simulink model "AOs_sim"  (R2024a)
settings: Solver=ode1  StartTime=0.0  StopTime=inf  FixedStep=0.002  RelTol=1e-3
(part 1 of 2)
settings Model: Creator=Enrica Tricomi  LastModifiedBy=tsmoragiewicz
settings OptimizationCC: ReuseModelBlockBuffer=off
settings RTWCC: GPUComputeCapability=3.5

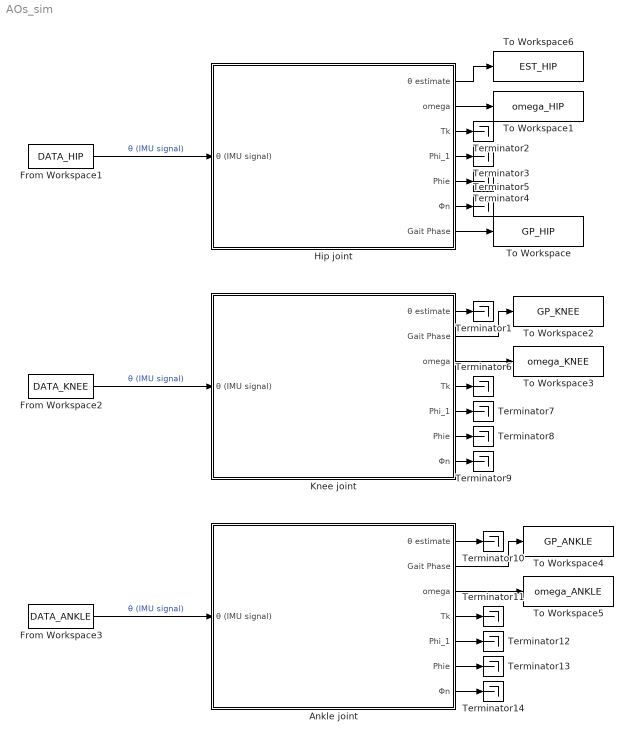
== system AOs_sim ==
  Ankle joint : Subsystem
  From Workspace1 : FromWorkspace  VariableName=DATA_HIP  SampleTime=-1
  From Workspace2 : FromWorkspace  VariableName=DATA_KNEE  SampleTime=-1
  From Workspace3 : FromWorkspace  VariableName=DATA_ANKLE  SampleTime=-1
  Hip joint : Subsystem
  Knee joint : Subsystem
  Terminator{1..14} (14 alike) : Terminator
  To Workspace : ToWorkspace  VariableName=GP_HIP  SampleTime=-1
  To Workspace1 : ToWorkspace  VariableName=omega_HIP  SampleTime=-1
  To Workspace2 : ToWorkspace  VariableName=GP_KNEE  SampleTime=-1
  To Workspace3 : ToWorkspace  VariableName=omega_KNEE  SampleTime=-1
  To Workspace4 : ToWorkspace  VariableName=GP_ANKLE  SampleTime=-1
  To Workspace5 : ToWorkspace  VariableName=omega_ANKLE  SampleTime=-1
  To Workspace6 : ToWorkspace  VariableName=EST_HIP  SampleTime=-1
  wires:
  Hip joint/4(Phi_1) -> Terminator3/1
  Hip joint/3(Tk) -> Terminator2/1
  Hip joint/1(θ estimate) -> To Workspace6/1
  Hip joint/6(Φn) -> Terminator5/1
  Hip joint/7(Gait Phase) -> To Workspace/1
  Hip joint/5(Phie) -> Terminator4/1
  Hip joint/2(omega) -> To Workspace1/1
  From Workspace1/1 -> Hip joint/1(θ (IMU signal))  "θ (IMU signal)"
  Knee joint/5(Phi_1) -> Terminator7/1
  Knee joint/4(Tk) -> Terminator6/1
  Knee joint/7(Φn) -> Terminator9/1
  Knee joint/2(Gait Phase) -> To Workspace2/1
  Knee joint/6(Phie) -> Terminator8/1
  Knee joint/3(omega) -> To Workspace3/1
  Knee joint/1(θ estimate) -> Terminator1/1
  Ankle joint/2(Gait Phase) -> To Workspace4/1
  Ankle joint/3(omega) -> To Workspace5/1
  Ankle joint/6(Phie) -> Terminator13/1
  Ankle joint/7(Φn) -> Terminator14/1
  Ankle joint/4(Tk) -> Terminator11/1
  Ankle joint/5(Phi_1) -> Terminator12/1
  Ankle joint/1(θ estimate) -> Terminator10/1
  From Workspace3/1 -> Ankle joint/1(θ (IMU signal))  "θ (IMU signal)"
  From Workspace2/1 -> Knee joint/1(θ (IMU signal))  "θ (IMU signal)"

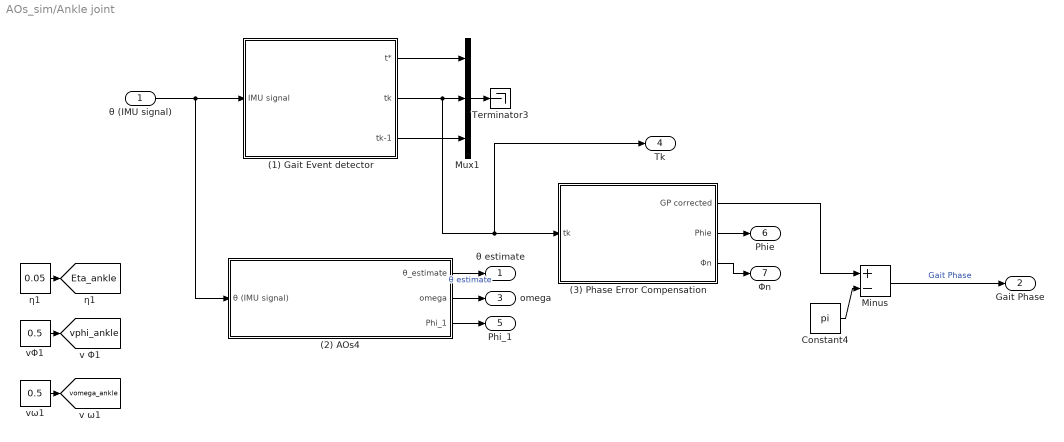
== system AOs_sim/Ankle joint ==
  θ (IMU signal) : Inport
  (1) Gait Event detector : Subsystem
  (2) AOs4 : Subsystem
  (3) Phase Error Compensation : Subsystem
  Constant4 : Constant  Value=pi
  Minus : Sum  Inputs=+-
  Mux1 : Mux  Inputs=3
  Terminator3 : Terminator
  vΦ1 : Constant  Value=0.5
  vω1 : Constant  Value=0.5
  η1 : Constant  Value=0.05
  θ estimate : Outport
  Gait Phase : Outport  Port=2
  omega : Outport  Port=3
  Tk : Outport  Port=4
  Phi_1 : Outport  Port=5
  Phie : Outport  Port=6
  Φn : Outport  Port=7
  tag scope: Eta_ankle=global, vomega_ankle=global, vphi_ankle=global
  wires:
  Constant4/1 -> Minus/2
  Mux1/1 -> Terminator3/1
  (2) AOs4/1(θ_estimate) -> θ estimate/1  "θ estimate"
  (1) Gait Event detector/3(tk-1) -> Mux1/3
  (1) Gait Event detector/1(t*) -> Mux1/1
  θ (IMU signal)/1 -> (1) Gait Event detector/1(IMU signal), (2) AOs4/1(θ (IMU signal))
  (3) Phase Error Compensation/1(GP corrected) -> Minus/1
  Minus/1 -> Gait Phase/1  "Gait Phase"
  (2) AOs4/2(omega) -> omega/1
  (1) Gait Event detector/2(tk) -> Tk/1, (3) Phase Error Compensation/1(tk), Mux1/2
  (2) AOs4/3(Phi_1) -> Phi_1/1
  (3) Phase Error Compensation/2(Phie) -> Phie/1
  (3) Phase Error Compensation/3(Φn) -> Φn/1
  vΦ1/1 -> [vphi_ankle]
  vω1/1 -> [vomega_ankle]
  η1/1 -> [Eta_ankle]

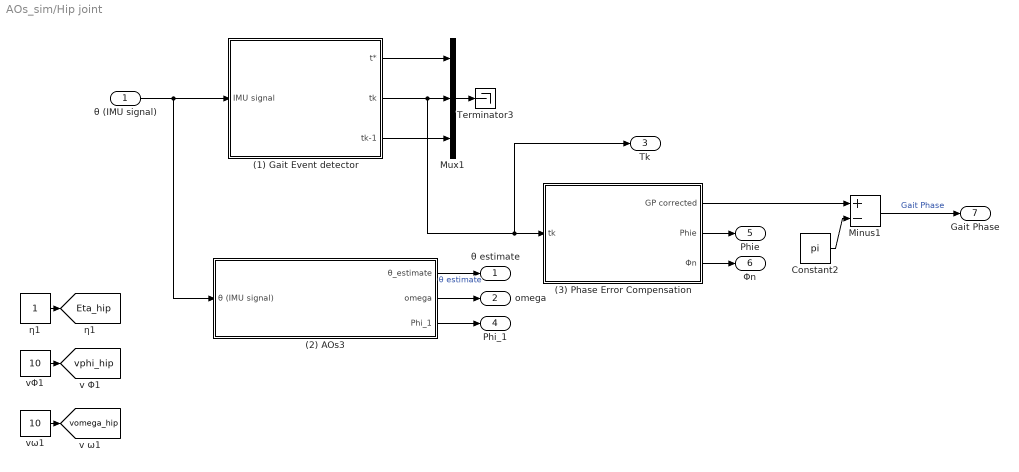
== system AOs_sim/Hip joint ==
  θ (IMU signal) : Inport
  (1) Gait Event detector : Subsystem
  (2) AOs3 : Subsystem
  (3) Phase Error Compensation : Subsystem
  Constant2 : Constant  Value=pi
  Minus1 : Sum  Inputs=+-
  Mux1 : Mux  Inputs=3
  Terminator3 : Terminator
  vΦ1 : Constant  Value=10
  vω1 : Constant  Value=10
  η1 : Constant
  θ estimate : Outport
  omega : Outport  Port=2
  Tk : Outport  Port=3
  Phi_1 : Outport  Port=4
  Phie : Outport  Port=5
  Φn : Outport  Port=6
  Gait Phase : Outport  Port=7
  tag scope: Eta_hip=global, vomega_hip=global, vphi_hip=global
  wires:
  Mux1/1 -> Terminator3/1
  (2) AOs3/1(θ_estimate) -> θ estimate/1  "θ estimate"
  (1) Gait Event detector/3(tk-1) -> Mux1/3
  (1) Gait Event detector/1(t*) -> Mux1/1
  (2) AOs3/2(omega) -> omega/1
  (1) Gait Event detector/2(tk) -> Tk/1, (3) Phase Error Compensation/1(tk), Mux1/2
  (3) Phase Error Compensation/2(Phie) -> Phie/1
  (3) Phase Error Compensation/3(Φn) -> Φn/1
  (2) AOs3/3(Phi_1) -> Phi_1/1
  Constant2/1 -> Minus1/2
  (3) Phase Error Compensation/1(GP corrected) -> Minus1/1
  Minus1/1 -> Gait Phase/1  "Gait Phase"
  θ (IMU signal)/1 -> (1) Gait Event detector/1(IMU signal), (2) AOs3/1(θ (IMU signal))
  vΦ1/1 -> [vphi_hip]
  vω1/1 -> [vomega_hip]
  η1/1 -> [Eta_hip]

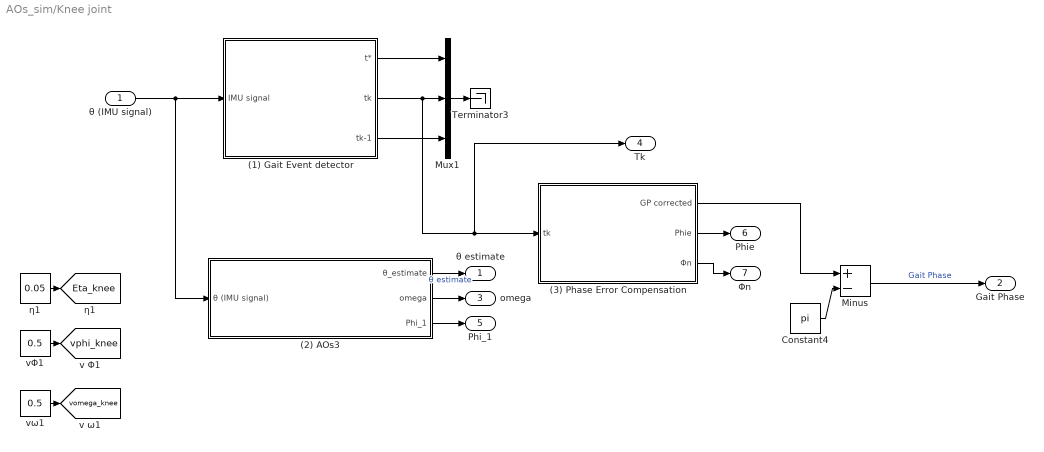
== system AOs_sim/Knee joint ==
  θ (IMU signal) : Inport
  (1) Gait Event detector : Subsystem
  (2) AOs3 : Subsystem
  (3) Phase Error Compensation : Subsystem
  Constant4 : Constant  Value=pi
  Minus : Sum  Inputs=+-
  Mux1 : Mux  Inputs=3
  Terminator3 : Terminator
  vΦ1 : Constant  Value=0.5
  vω1 : Constant  Value=0.5
  η1 : Constant  Value=0.05
  θ estimate : Outport
  Gait Phase : Outport  Port=2
  omega : Outport  Port=3
  Tk : Outport  Port=4
  Phi_1 : Outport  Port=5
  Phie : Outport  Port=6
  Φn : Outport  Port=7
  tag scope: Eta_knee=global, vomega_knee=global, vphi_knee=global
  wires:
  Constant4/1 -> Minus/2
  Mux1/1 -> Terminator3/1
  (2) AOs3/1(θ_estimate) -> θ estimate/1  "θ estimate"
  (1) Gait Event detector/3(tk-1) -> Mux1/3
  (1) Gait Event detector/1(t*) -> Mux1/1
  θ (IMU signal)/1 -> (1) Gait Event detector/1(IMU signal), (2) AOs3/1(θ (IMU signal))
  (3) Phase Error Compensation/1(GP corrected) -> Minus/1
  Minus/1 -> Gait Phase/1  "Gait Phase"
  (2) AOs3/2(omega) -> omega/1
  (1) Gait Event detector/2(tk) -> Tk/1, (3) Phase Error Compensation/1(tk), Mux1/2
  (2) AOs3/3(Phi_1) -> Phi_1/1
  (3) Phase Error Compensation/2(Phie) -> Phie/1
  (3) Phase Error Compensation/3(Φn) -> Φn/1
  η1/1 -> [Eta_knee]
  vω1/1 -> [vomega_knee]
  vΦ1/1 -> [vphi_knee]

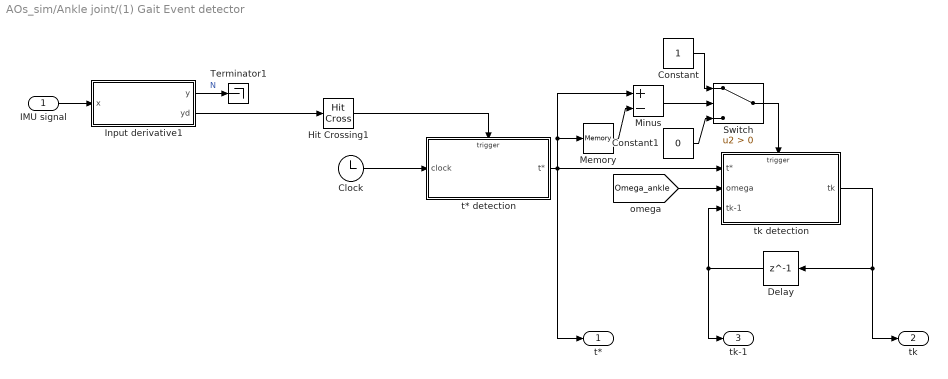
== system AOs_sim/Ankle joint/(1) Gait Event detector ==
  IMU signal : Inport
  Clock : Clock
  Constant : Constant
  Constant1 : Constant  Value=0
  Delay : Delay  DelayLength=1
  Hit Crossing1 : HitCross  HitCrossingOffset=0.2  HitCrossingDirection=falling
  Input derivative1 : Subsystem  mask{wn=40, zt=1, x0=0}
      mask prompts: wn "Cut-off frequency (rad/s)"; zt "Damping ratio"; x0 "Initial Condition"
      mask Display: disp('Second-Order\nLow-Pass Filter');
  Memory : Memory
  Minus : Sum  Inputs=+-
  Switch : Switch  Criteria=u2 > Threshold  SaturateOnIntegerOverflow=off  InputSameDT=off
  Terminator1 : Terminator
  t* detection : Subsystem
  tk detection : Subsystem
  t* : Outport
  tk : Outport  Port=2
  tk-1 : Outport  Port=3
  wires:
  Clock/1 -> t* detection/1(clock)
  Hit Crossing1/1 -> t* detection/Trigger
  t* detection/1(t*) -> tk detection/1(t*), t*/1, Minus/1, Memory/1
  [Omega_ankle] -> tk detection/2(omega)
  Constant/1 -> Switch/1
  Constant1/1 -> Switch/3
  Minus/1 -> Switch/2
  Memory/1 -> Minus/2
  Switch/1 -> tk detection/Trigger
  Delay/1 -> tk detection/3(tk-1), tk-1/1
  tk detection/1(tk) -> tk/1, Delay/1
  Input derivative1/2(yd) -> Hit Crossing1/1
  IMU signal/1 -> Input derivative1/1(x)
  Input derivative1/1(y) -> Terminator1/1  "N"

== system AOs_sim/Ankle joint/(2) AOs4 ==
  note: Pool of Adaptive Oscillators
  θ (IMU signal) : Inport
  AO0 : Subsystem
  AO1 : Subsystem
  AO2 : Subsystem
  AO3 : Subsystem
  AO4 : Subsystem
  AO5 : Subsystem
  Sum : Sum  Inputs=|+-
  Sum1 : Sum  Inputs=6
  θ_estimate : Outport
  omega : Outport  Port=2
  Phi_1 : Outport  Port=3
  tag scope: Ft_ankle=global
  wires:
  AO0/1(α0) -> Sum1/1
  Sum1/1 -> θ_estimate/1, Sum/2  "θ_estimate"
  AO4/1(θ_est3) -> Sum1/6
  AO1/1(θ_est1) -> Sum1/2
  Sum/1 -> [Ft_ankle]
  AO2/1(θ_est2) -> Sum1/3
  θ (IMU signal)/1 -> Sum/1
  AO4/2(omega) -> omega/1
  AO1/2(Phi_1) -> Phi_1/1
  AO3/1(θ_est2) -> Sum1/4
  AO5/1(θ_est2) -> Sum1/5

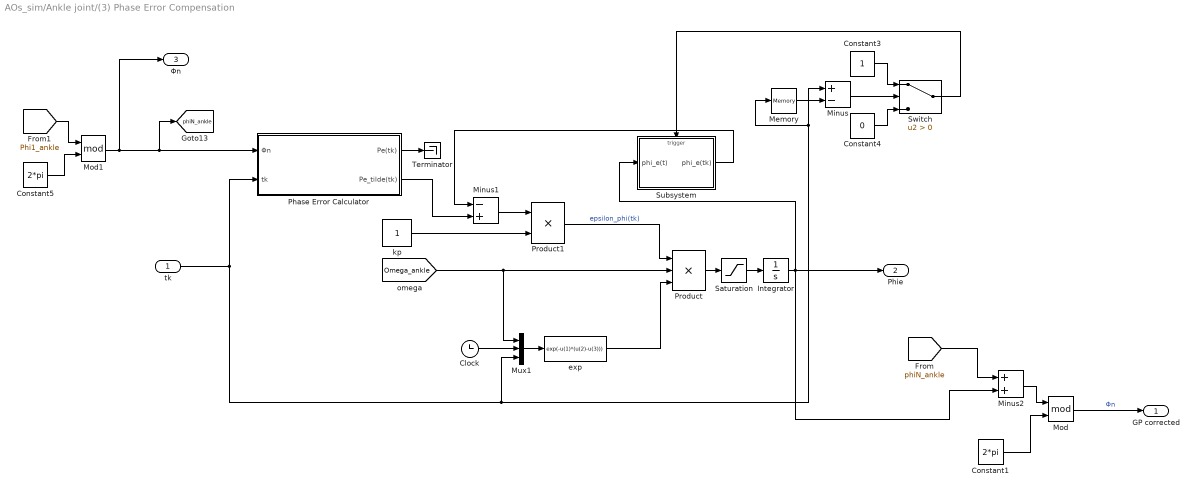
== system AOs_sim/Ankle joint/(3) Phase Error Compensation ==
  tk : Inport
  Clock : Clock
  Constant1 : Constant  Value=2*pi
  Constant3 : Constant
  Constant4 : Constant  Value=0
  Constant5 : Constant  Value=2*pi
  Integrator : Integrator  InitialCondition=0.01
  Memory : Memory
  Minus : Sum  Inputs=+-
  Minus1 : Sum  Inputs=-+
  Minus2 : Sum
  Mod : Math  Operator=mod
  Mod1 : Math  Operator=mod
  Mux1 : Mux  Inputs=3
  Phase Error Calculator : Subsystem
  Product : Product  Inputs=3
  Product1 : Product
  Saturation : Saturate  UpperLimit=10^10  LowerLimit=-10^10
  Subsystem : Subsystem
  Switch : Switch  Criteria=u2 > Threshold  SaturateOnIntegerOverflow=off  InputSameDT=off
  Terminator : Terminator
  exp : Fcn  Expr=exp(-u(1)*(u(2)-u(3)))
  kp : Constant
  GP corrected : Outport
  Phie : Outport  Port=2
  Φn : Outport  Port=3
  tag scope: phiN_ankle=global
  wires:
  Integrator/1 -> Minus2/2, Phie/1, Subsystem/1(phi_e(t))
  Constant1/1 -> Mod/2
  Mux1/1 -> exp/1
  Clock/1 -> Mux1/2
  [phiN_ankle] -> Minus2/1
  [Phi1_ankle] -> Mod1/1
  Product/1 -> Saturation/1
  Minus2/1 -> Mod/1
  Minus1/1 -> Product1/1
  kp/1 -> Product1/2
  Product1/1 -> Product/1  "epsilon_phi(tk)"
  Phase Error Calculator/2(Pe_tilde(tk)) -> Minus1/2
  [Omega_ankle] -> Mux1/1, Product/2
  exp/1 -> Product/3
  Saturation/1 -> Integrator/1
  Constant3/1 -> Switch/1
  Memory/1 -> Minus/2
  Constant4/1 -> Switch/3
  Minus/1 -> Switch/2
  tk/1 -> Phase Error Calculator/2(tk), Minus/1, Memory/1, Mux1/3
  Switch/1 -> Subsystem/Trigger
  Subsystem/1(phi_e(tk)) -> Minus1/1
  Constant5/1 -> Mod1/2
  Mod/1 -> GP corrected/1  "Φn"
  Mod1/1 -> Φn/1, [phiN_ankle], Phase Error Calculator/1(Φn)
  Phase Error Calculator/1(Pe(tk)) -> Terminator/1

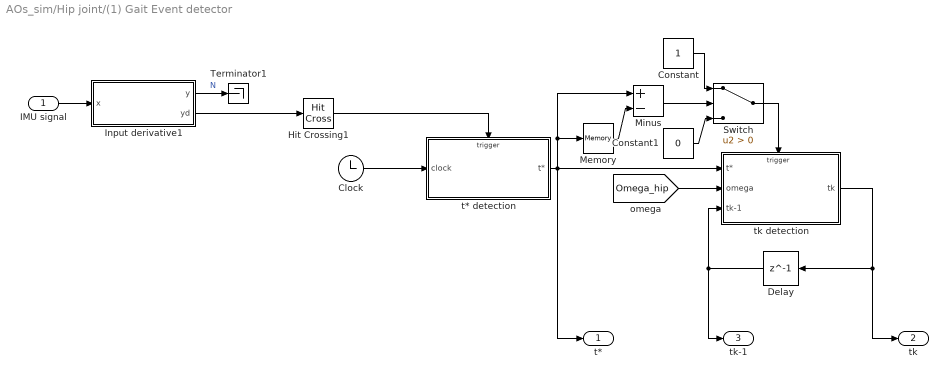
== system AOs_sim/Hip joint/(1) Gait Event detector ==
  IMU signal : Inport
  Clock : Clock
  Constant : Constant
  Constant1 : Constant  Value=0
  Delay : Delay  DelayLength=1
  Hit Crossing1 : HitCross  HitCrossingOffset=0.2  HitCrossingDirection=falling
  Input derivative1 : Subsystem  mask{wn=40, zt=1, x0=0}
      mask prompts: wn "Cut-off frequency (rad/s)"; zt "Damping ratio"; x0 "Initial Condition"
      mask Display: disp('Second-Order\nLow-Pass Filter');
  Memory : Memory
  Minus : Sum  Inputs=+-
  Switch : Switch  Criteria=u2 > Threshold  SaturateOnIntegerOverflow=off  InputSameDT=off
  Terminator1 : Terminator
  t* detection : Subsystem
  tk detection : Subsystem
  t* : Outport
  tk : Outport  Port=2
  tk-1 : Outport  Port=3
  wires:
  Clock/1 -> t* detection/1(clock)
  Hit Crossing1/1 -> t* detection/Trigger
  t* detection/1(t*) -> tk detection/1(t*), t*/1, Minus/1, Memory/1
  [Omega_hip] -> tk detection/2(omega)
  Constant/1 -> Switch/1
  Constant1/1 -> Switch/3
  Minus/1 -> Switch/2
  Memory/1 -> Minus/2
  Switch/1 -> tk detection/Trigger
  Delay/1 -> tk detection/3(tk-1), tk-1/1
  tk detection/1(tk) -> tk/1, Delay/1
  Input derivative1/2(yd) -> Hit Crossing1/1
  IMU signal/1 -> Input derivative1/1(x)
  Input derivative1/1(y) -> Terminator1/1  "N"

== system AOs_sim/Hip joint/(2) AOs3 ==
  note: Pool of Adaptive Oscillators
  θ (IMU signal) : Inport
  AO0 : Subsystem
  AO1 : Subsystem
  AO2 : Subsystem
  AO3 : Subsystem
  Sum : Sum  Inputs=|+-
  Sum1 : Sum  Inputs=4
  θ_estimate : Outport
  omega : Outport  Port=2
  Phi_1 : Outport  Port=3
  tag scope: Ft_hip=global
  wires:
  AO0/1(α0) -> Sum1/1
  Sum1/1 -> θ_estimate/1, Sum/2  "θ_estimate"
  AO3/1(θ_est3) -> Sum1/4
  AO1/1(θ_est1) -> Sum1/2
  Sum/1 -> [Ft_hip]
  AO2/1(θ_est2) -> Sum1/3
  θ (IMU signal)/1 -> Sum/1
  AO3/2(omega) -> omega/1
  AO1/2(Phi_1) -> Phi_1/1

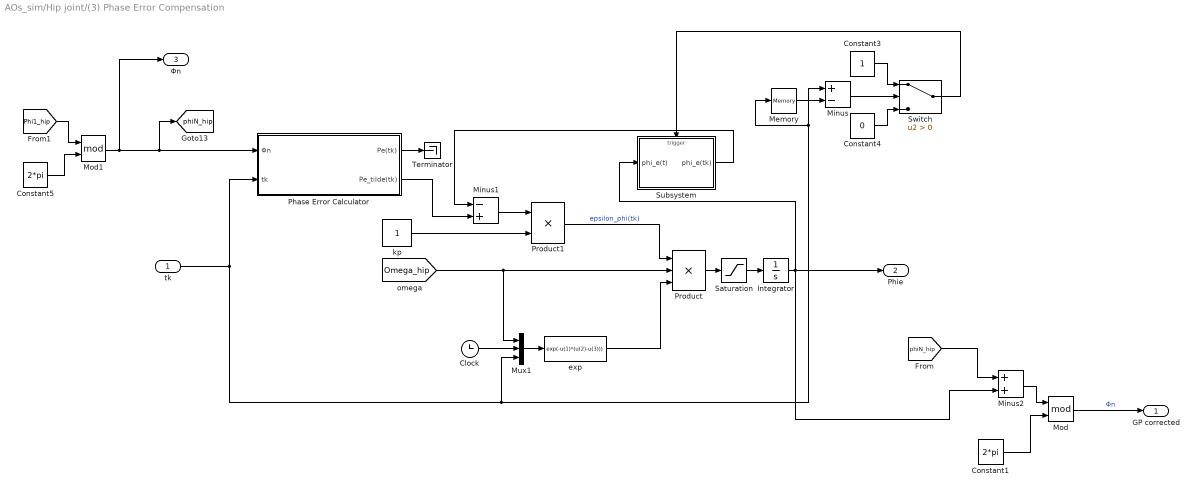
== system AOs_sim/Hip joint/(3) Phase Error Compensation ==
  tk : Inport
  Clock : Clock
  Constant1 : Constant  Value=2*pi
  Constant3 : Constant
  Constant4 : Constant  Value=0
  Constant5 : Constant  Value=2*pi
  Integrator : Integrator  InitialCondition=0.01
  Memory : Memory
  Minus : Sum  Inputs=+-
  Minus1 : Sum  Inputs=-+
  Minus2 : Sum
  Mod : Math  Operator=mod
  Mod1 : Math  Operator=mod
  Mux1 : Mux  Inputs=3
  Phase Error Calculator : Subsystem
  Product : Product  Inputs=3
  Product1 : Product
  Saturation : Saturate  UpperLimit=10^10  LowerLimit=-10^10
  Subsystem : Subsystem
  Switch : Switch  Criteria=u2 > Threshold  SaturateOnIntegerOverflow=off  InputSameDT=off
  Terminator : Terminator
  exp : Fcn  Expr=exp(-u(1)*(u(2)-u(3)))
  kp : Constant
  GP corrected : Outport
  Phie : Outport  Port=2
  Φn : Outport  Port=3
  tag scope: phiN_hip=global
  wires:
  Integrator/1 -> Minus2/2, Phie/1, Subsystem/1(phi_e(t))
  Constant1/1 -> Mod/2
  Mux1/1 -> exp/1
  Clock/1 -> Mux1/2
  [phiN_hip] -> Minus2/1
  [Phi1_hip] -> Mod1/1
  Product/1 -> Saturation/1
  Minus2/1 -> Mod/1
  Minus1/1 -> Product1/1
  kp/1 -> Product1/2
  Product1/1 -> Product/1  "epsilon_phi(tk)"
  Phase Error Calculator/2(Pe_tilde(tk)) -> Minus1/2
  [Omega_hip] -> Mux1/1, Product/2
  exp/1 -> Product/3
  Saturation/1 -> Integrator/1
  Constant3/1 -> Switch/1
  Memory/1 -> Minus/2
  Constant4/1 -> Switch/3
  Minus/1 -> Switch/2
  tk/1 -> Phase Error Calculator/2(tk), Minus/1, Memory/1, Mux1/3
  Switch/1 -> Subsystem/Trigger
  Subsystem/1(phi_e(tk)) -> Minus1/1
  Constant5/1 -> Mod1/2
  Mod/1 -> GP corrected/1  "Φn"
  Mod1/1 -> Φn/1, [phiN_hip], Phase Error Calculator/1(Φn)
  Phase Error Calculator/1(Pe(tk)) -> Terminator/1

== system AOs_sim/Knee joint/(1) Gait Event detector ==
  IMU signal : Inport
  Clock : Clock
  Constant : Constant
  Constant1 : Constant  Value=0
  Delay : Delay  DelayLength=1
  Hit Crossing1 : HitCross  HitCrossingOffset=0.2  HitCrossingDirection=falling
  Input derivative1 : Subsystem  mask{wn=40, zt=1, x0=0}
      mask prompts: wn "Cut-off frequency (rad/s)"; zt "Damping ratio"; x0 "Initial Condition"
      mask Display: disp('Second-Order\nLow-Pass Filter');
  Memory : Memory
  Minus : Sum  Inputs=+-
  Switch : Switch  Criteria=u2 > Threshold  SaturateOnIntegerOverflow=off  InputSameDT=off
  Terminator1 : Terminator
  t* detection : Subsystem
  tk detection : Subsystem
  t* : Outport
  tk : Outport  Port=2
  tk-1 : Outport  Port=3
  wires:
  Clock/1 -> t* detection/1(clock)
  Hit Crossing1/1 -> t* detection/Trigger
  t* detection/1(t*) -> tk detection/1(t*), t*/1, Minus/1, Memory/1
  [Omega_knee] -> tk detection/2(omega)
  Constant/1 -> Switch/1
  Constant1/1 -> Switch/3
  Minus/1 -> Switch/2
  Memory/1 -> Minus/2
  Switch/1 -> tk detection/Trigger
  Delay/1 -> tk detection/3(tk-1), tk-1/1
  tk detection/1(tk) -> tk/1, Delay/1
  Input derivative1/2(yd) -> Hit Crossing1/1
  IMU signal/1 -> Input derivative1/1(x)
  Input derivative1/1(y) -> Terminator1/1  "N"

== system AOs_sim/Knee joint/(2) AOs3 ==
  note: Pool of Adaptive Oscillators
  θ (IMU signal) : Inport
  AO0 : Subsystem
  AO1 : Subsystem
  AO2 : Subsystem
  AO3 : Subsystem
  AO4 : Subsystem
  Sum : Sum  Inputs=|+-
  Sum1 : Sum  Inputs=5
  θ_estimate : Outport
  omega : Outport  Port=2
  Phi_1 : Outport  Port=3
  tag scope: Ft_knee=global
  wires:
  AO0/1(α0) -> Sum1/1
  Sum1/1 -> Sum/2, θ_estimate/1  "θ_estimate"
  AO4/1(θ_est3) -> Sum1/5
  AO1/1(θ_est1) -> Sum1/2
  Sum/1 -> [Ft_knee]
  AO2/1(θ_est2) -> Sum1/3
  θ (IMU signal)/1 -> Sum/1
  AO4/2(omega) -> omega/1
  AO1/2(Phi_1) -> Phi_1/1
  AO3/1(θ_est2) -> Sum1/4

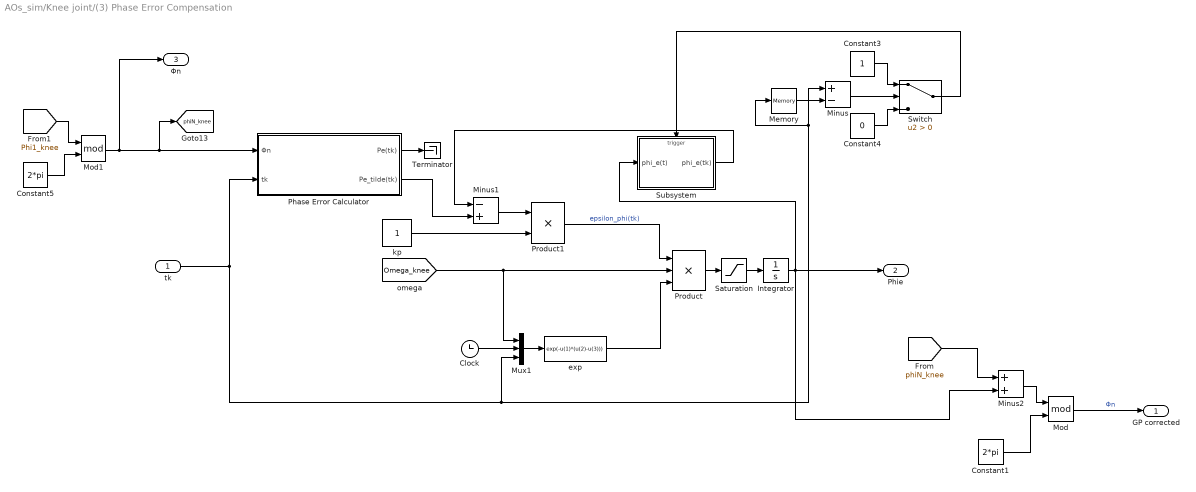
== system AOs_sim/Knee joint/(3) Phase Error Compensation ==
  tk : Inport
  Clock : Clock
  Constant1 : Constant  Value=2*pi
  Constant3 : Constant
  Constant4 : Constant  Value=0
  Constant5 : Constant  Value=2*pi
  Integrator : Integrator  InitialCondition=0.01
  Memory : Memory
  Minus : Sum  Inputs=+-
  Minus1 : Sum  Inputs=-+
  Minus2 : Sum
  Mod : Math  Operator=mod
  Mod1 : Math  Operator=mod
  Mux1 : Mux  Inputs=3
  Phase Error Calculator : Subsystem
  Product : Product  Inputs=3
  Product1 : Product
  Saturation : Saturate  UpperLimit=10^10  LowerLimit=-10^10
  Subsystem : Subsystem
  Switch : Switch  Criteria=u2 > Threshold  SaturateOnIntegerOverflow=off  InputSameDT=off
  Terminator : Terminator
  exp : Fcn  Expr=exp(-u(1)*(u(2)-u(3)))
  kp : Constant
  GP corrected : Outport
  Phie : Outport  Port=2
  Φn : Outport  Port=3
  tag scope: phiN_knee=global
  wires:
  Integrator/1 -> Minus2/2, Phie/1, Subsystem/1(phi_e(t))
  Constant1/1 -> Mod/2
  Mux1/1 -> exp/1
  Clock/1 -> Mux1/2
  [phiN_knee] -> Minus2/1
  [Phi1_knee] -> Mod1/1
  Product/1 -> Saturation/1
  Minus2/1 -> Mod/1
  Minus1/1 -> Product1/1
  kp/1 -> Product1/2
  Product1/1 -> Product/1  "epsilon_phi(tk)"
  Phase Error Calculator/2(Pe_tilde(tk)) -> Minus1/2
  [Omega_knee] -> Mux1/1, Product/2
  exp/1 -> Product/3
  Saturation/1 -> Integrator/1
  Constant3/1 -> Switch/1
  Memory/1 -> Minus/2
  Constant4/1 -> Switch/3
  Minus/1 -> Switch/2
  tk/1 -> Phase Error Calculator/2(tk), Minus/1, Memory/1, Mux1/3
  Switch/1 -> Subsystem/Trigger
  Subsystem/1(phi_e(tk)) -> Minus1/1
  Constant5/1 -> Mod1/2
  Mod/1 -> GP corrected/1  "Φn"
  Mod1/1 -> Φn/1, [phiN_knee], Phase Error Calculator/1(Φn)
  Phase Error Calculator/1(Pe(tk)) -> Terminator/1

== system AOs_sim/Ankle joint/(1) Gait Event detector/Input derivative1 ==
  x : Inport
  Constant : Constant  Value=2
  Integrator1 : Integrator  InitialConditionSource=external
  Integrator2 : Integrator
  Product : Product  RndMeth=Zero
  Product1 : Product  RndMeth=Zero
  Product2 : Product  Inputs=3  RndMeth=Zero
  Sum : Sum  Inputs=|+-
  Sum1 : Sum  Inputs=|+-
  wn : Constant  Value=wn
  x0 : Constant  Value=x0
  zt : Constant  Value=zt
  y : Outport  VectorParamsAs1DForOutWhenUnconnected=off
  yd : Outport  Port=2  VectorParamsAs1DForOutWhenUnconnected=off
  wires:
  Sum/1 -> Product/2
  wn/1 -> Product/1, Product1/1
  Sum1/1 -> Sum/1
  x0/1 -> Integrator1/2
  Integrator2/1 -> Product1/2, Product2/1
  Product/1 -> Integrator2/1
  x/1 -> Sum1/1
  Product1/1 -> Integrator1/1, yd/1
  Integrator1/1 -> Sum1/2, y/1
  Product2/1 -> Sum/2
  zt/1 -> Product2/3
  Constant/1 -> Product2/2

== system AOs_sim/Ankle joint/(1) Gait Event detector/t* detection ==
  clock : Inport
  Trigger : TriggerPort  VariantControl=Variant  PortDimensions=1
  t* : Outport
  wires:
  clock/1 -> t*/1

== system AOs_sim/Ankle joint/(1) Gait Event detector/tk detection ==
  t* : Inport
  omega : Inport  Port=2
  tk-1 : Inport  Port=3
  Trigger : TriggerPort  VariantControl=Variant  PortDimensions=1
  Constant2 : Constant  Value=eps
  Constant3 : Constant  Value=2*pi
  Constant4 : Constant
  Constant5 : Constant  Value=0
  Divide : Product  Inputs=*/
  Minus : Sum  Inputs=+--
  Sum : Sum  Inputs=|++
  Switch1 : Switch  SaturateOnIntegerOverflow=off  InputSameDT=off
  ro : Gain  Gain=0.7
  tk+1 detection : Subsystem
  tk : Outport
  wires:
  Constant5/1 -> Switch1/3
  Sum/1 -> Divide/2
  Constant3/1 -> Divide/1
  Constant4/1 -> Switch1/1
  Constant2/1 -> Sum/2
  Divide/1 -> ro/1  "T(t)"
  t*/1 -> Minus/1, tk+1 detection/1(t*)
  tk-1/1 -> Minus/3
  ro/1 -> Minus/2
  tk+1 detection/1(tk) -> tk/1
  Switch1/1 -> tk+1 detection/Enable
  Minus/1 -> Switch1/2
  omega/1 -> Sum/1

== system AOs_sim/Ankle joint/(2) AOs4/AO0 ==
  Integrator1 : Integrator  InitialCondition=0.01
  Product : Product
  α0 : Outport
  tag scope: Alpha0_ankle=global
  wires:
  Product/1 -> Integrator1/1  "α0_dot(t)"
  [Eta_ankle] -> Product/1
  [Ft_ankle] -> Product/2
  Integrator1/1 -> [Alpha0_ankle], α0/1  "α0(t)"

== system AOs_sim/Ankle joint/(2) AOs4/AO1 ==
  Integrator : Integrator  ContinuousStateAttributes='Phase'
  Integrator1 : Integrator  ContinuousStateAttributes='Amplitude'
  Mux : Mux  Inputs=2
  Mux1 : Mux  Inputs=2
  Φ1_dot(t) : Subsystem
  α_dot(t) : Subsystem
  θ_estimated : Fcn  Expr=u(1)*sin(u(2))
  θ_est1 : Outport
  Phi_1 : Outport  Port=2
  tag scope: Alpha1_ankle=global, Phi1_ankle=global
  wires:
  Integrator/1 -> Mux/2, Phi_1/1, [Phi1_ankle], Mux1/2  "Φ1(t)"
  Mux/1 -> Φ1_dot(t)/1(In1), α_dot(t)/1(Input)
  Integrator1/1 -> Mux/1, [Alpha1_ankle], Mux1/1  "α1(t)"
  Mux1/1 -> θ_estimated/1
  θ_estimated/1 -> θ_est1/1  "θ_estimated"
  α_dot(t)/1(α_dot(t)) -> Integrator1/1
  Φ1_dot(t)/1(Φ1_dot(t)) -> Integrator/1

== system AOs_sim/Ankle joint/(2) AOs4/AO2 ==
  Integrator : Integrator  ContinuousStateAttributes='Phase'
  Integrator1 : Integrator  ContinuousStateAttributes='Amplitude'
  Mux : Mux  Inputs=2
  Mux1 : Mux  Inputs=2
  Φ2_dot(t) : Subsystem
  α_dot(t) : Subsystem
  θ_estimated : Fcn  Expr=u(1)*sin(u(2))
  θ_est2 : Outport
  tag scope: Alpha2_ankle=global
  wires:
  Integrator/1 -> Mux/2, Mux1/2  "Φ2(t)"
  Mux/1 -> Φ2_dot(t)/1(In1), α_dot(t)/1(Input)
  Integrator1/1 -> Mux/1, [Alpha2_ankle], Mux1/1  "α2(t)"
  Mux1/1 -> θ_estimated/1
  θ_estimated/1 -> θ_est2/1  "θ_estimated"
  α_dot(t)/1(α_dot(t)) -> Integrator1/1
  Φ2_dot(t)/1(Φ2_dot(t)) -> Integrator/1

== system AOs_sim/Ankle joint/(2) AOs4/AO3 ==
  Integrator : Integrator  ContinuousStateAttributes='Phase'
  Integrator1 : Integrator  ContinuousStateAttributes='Amplitude'
  Mux : Mux  Inputs=2
  Mux1 : Mux  Inputs=2
  Φ2_dot(t) : Subsystem
  α_dot(t) : Subsystem
  θ_estimated : Fcn  Expr=u(1)*sin(u(2))
  θ_est2 : Outport
  tag scope: Alpha3_ankle=global
  wires:
  Integrator/1 -> Mux/2, Mux1/2  "Φ2(t)"
  Mux/1 -> Φ2_dot(t)/1(In1), α_dot(t)/1(Input)
  Integrator1/1 -> Mux/1, [Alpha3_ankle], Mux1/1  "α2(t)"
  Mux1/1 -> θ_estimated/1
  θ_estimated/1 -> θ_est2/1  "θ_estimated"
  α_dot(t)/1(α_dot(t)) -> Integrator1/1
  Φ2_dot(t)/1(Φ2_dot(t)) -> Integrator/1

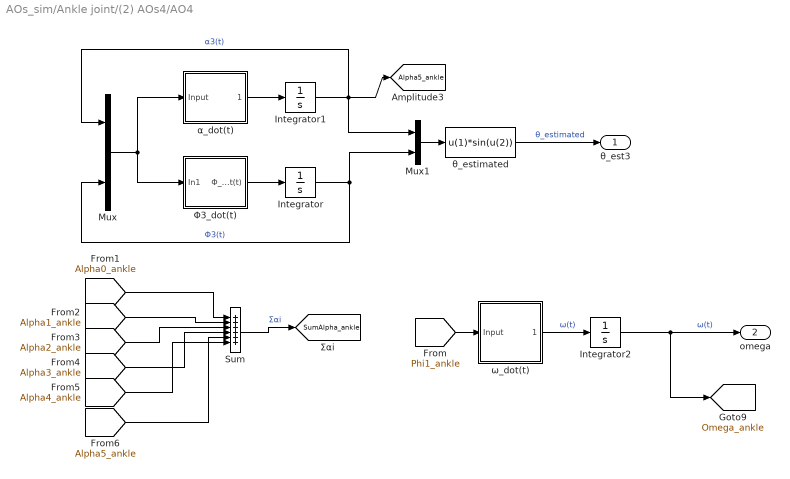
== system AOs_sim/Ankle joint/(2) AOs4/AO4 ==
  Integrator : Integrator  ContinuousStateAttributes='Phase'
  Integrator1 : Integrator  ContinuousStateAttributes='Amplitude'
  Integrator2 : Integrator  WrapState=on  WrappedStateUpperValue=10*pi  WrappedStateLowerValue=0  ContinuousStateAttributes='Omega'
  Mux : Mux  Inputs=2
  Mux1 : Mux  Inputs=2
  Sum : Sum  Inputs=++++++
  Φ3_dot(t) : Subsystem
  α_dot(t) : Subsystem
  θ_estimated : Fcn  Expr=u(1)*sin(u(2))
  ω_dot(t) : Subsystem
  θ_est3 : Outport
  omega : Outport  Port=2
  tag scope: Alpha5_ankle=global, Omega_ankle=global, SumAlpha_ankle=global
  wires:
  θ_estimated/1 -> θ_est3/1  "θ_estimated"
  α_dot(t)/1(α_dot(t)) -> Integrator1/1
  Integrator/1 -> Mux/2, Mux1/2  "Φ3(t)"
  Mux1/1 -> θ_estimated/1
  Φ3_dot(t)/1(Φ_dot(t)) -> Integrator/1
  Integrator1/1 -> Mux/1, [Alpha5_ankle], Mux1/1  "α3(t)"
  Mux/1 -> Φ3_dot(t)/1(In1), α_dot(t)/1(Input)
  [Alpha1_ankle] -> Sum/2
  [Alpha2_ankle] -> Sum/3
  Sum/1 -> [SumAlpha_ankle]  "Σαi"
  [Alpha3_ankle] -> Sum/4
  [Alpha0_ankle] -> Sum/1
  ω_dot(t)/1(ω_dot(t)) -> Integrator2/1  "ω(t)"
  [Phi1_ankle] -> ω_dot(t)/1(Input)
  Integrator2/1 -> [Omega_ankle], omega/1  "ω(t)"
  [Alpha4_ankle] -> Sum/6
  [Alpha5_ankle] -> Sum/5

== system AOs_sim/Ankle joint/(2) AOs4/AO5 ==
  Integrator : Integrator  ContinuousStateAttributes='Phase'
  Integrator1 : Integrator  ContinuousStateAttributes='Amplitude'
  Mux : Mux  Inputs=2
  Mux1 : Mux  Inputs=2
  Φ2_dot(t) : Subsystem
  α_dot(t) : Subsystem
  θ_estimated : Fcn  Expr=u(1)*sin(u(2))
  θ_est2 : Outport
  tag scope: Alpha4_ankle=global
  wires:
  Integrator/1 -> Mux/2, Mux1/2  "Φ2(t)"
  Mux/1 -> Φ2_dot(t)/1(In1), α_dot(t)/1(Input)
  Integrator1/1 -> Mux/1, [Alpha4_ankle], Mux1/1  "α2(t)"
  Mux1/1 -> θ_estimated/1
  θ_estimated/1 -> θ_est2/1  "θ_estimated"
  α_dot(t)/1(α_dot(t)) -> Integrator1/1
  Φ2_dot(t)/1(Φ2_dot(t)) -> Integrator/1

== system AOs_sim/Ankle joint/(3) Phase Error Compensation/Phase Error Calculator ==
  Φn : Inport
  tk : Inport  Port=2
  Constant : Constant
  Constant2 : Constant  Value=0
  Delay : Delay  DelayLength=1
  Memory : Memory
  Minus : Sum  Inputs=+-
  Subsystem : Subsystem
  Subsystem1 : Subsystem
  Switch : Switch  Criteria=u2 > Threshold  SaturateOnIntegerOverflow=off  InputSameDT=off
  Pe(tk) : Outport
  Pe_tilde(tk) : Outport  Port=2
  wires:
  Subsystem/1(Pe(tk)) -> Pe(tk)/1
  tk/1 -> Memory/1, Minus/1
  Memory/1 -> Minus/2
  Minus/1 -> Switch/2
  Constant2/1 -> Switch/3
  Constant/1 -> Switch/1
  Subsystem/2(Pe_tilde(tk)) -> Pe_tilde(tk)/1, Delay/1
  Φn/1 -> Subsystem/1(Φn)
  Subsystem1/1(Pe_tilde(tk-1)) -> Subsystem/2(Pe_tilde(tk-1))
  Switch/1 -> Subsystem1/Trigger, Subsystem/Trigger
  Delay/1 -> Subsystem1/1(Pe_tilde(tk))

== system AOs_sim/Ankle joint/(3) Phase Error Compensation/Subsystem ==
  phi_e(t) : Inport
  Trigger : TriggerPort  VariantControl=Variant  PortDimensions=1
  phi_e(tk) : Outport
  wires:
  phi_e(t)/1 -> phi_e(tk)/1

== system AOs_sim/Hip joint/(1) Gait Event detector/Input derivative1 ==
  x : Inport
  Constant : Constant  Value=2
  Integrator1 : Integrator  InitialConditionSource=external
  Integrator2 : Integrator
  Product : Product  RndMeth=Zero
  Product1 : Product  RndMeth=Zero
  Product2 : Product  Inputs=3  RndMeth=Zero
  Sum : Sum  Inputs=|+-
  Sum1 : Sum  Inputs=|+-
  wn : Constant  Value=wn
  x0 : Constant  Value=x0
  zt : Constant  Value=zt
  y : Outport  VectorParamsAs1DForOutWhenUnconnected=off
  yd : Outport  Port=2  VectorParamsAs1DForOutWhenUnconnected=off
  wires:
  Sum/1 -> Product/2
  wn/1 -> Product/1, Product1/1
  Sum1/1 -> Sum/1
  x0/1 -> Integrator1/2
  Integrator2/1 -> Product1/2, Product2/1
  Product/1 -> Integrator2/1
  x/1 -> Sum1/1
  Product1/1 -> Integrator1/1, yd/1
  Integrator1/1 -> Sum1/2, y/1
  Product2/1 -> Sum/2
  zt/1 -> Product2/3
  Constant/1 -> Product2/2

== system AOs_sim/Hip joint/(1) Gait Event detector/t* detection ==
  clock : Inport
  Trigger : TriggerPort  VariantControl=Variant  PortDimensions=1
  t* : Outport
  wires:
  clock/1 -> t*/1

== system AOs_sim/Hip joint/(1) Gait Event detector/tk detection ==
  t* : Inport
  omega : Inport  Port=2
  tk-1 : Inport  Port=3
  Trigger : TriggerPort  VariantControl=Variant  PortDimensions=1
  Constant2 : Constant  Value=eps
  Constant3 : Constant  Value=2*pi
  Constant4 : Constant
  Constant5 : Constant  Value=0
  Divide : Product  Inputs=*/
  Minus : Sum  Inputs=+--
  Sum : Sum  Inputs=|++
  Switch1 : Switch  SaturateOnIntegerOverflow=off  InputSameDT=off
  ro : Gain  Gain=0.7
  tk+1 detection : Subsystem
  tk : Outport
  wires:
  Constant5/1 -> Switch1/3
  Sum/1 -> Divide/2
  Constant3/1 -> Divide/1
  Constant4/1 -> Switch1/1
  Constant2/1 -> Sum/2
  Divide/1 -> ro/1  "T(t)"
  t*/1 -> Minus/1, tk+1 detection/1(t*)
  tk-1/1 -> Minus/3
  ro/1 -> Minus/2
  tk+1 detection/1(tk) -> tk/1
  Switch1/1 -> tk+1 detection/Enable
  Minus/1 -> Switch1/2
  omega/1 -> Sum/1

== system AOs_sim/Hip joint/(2) AOs3/AO0 ==
  Integrator1 : Integrator  InitialCondition=0.01
  Product : Product
  α0 : Outport
  tag scope: Alpha0_hip=global
  wires:
  Product/1 -> Integrator1/1  "α0_dot(t)"
  [Eta_hip] -> Product/1
  [Ft_hip] -> Product/2
  Integrator1/1 -> [Alpha0_hip], α0/1  "α0(t)"

== system AOs_sim/Hip joint/(2) AOs3/AO1 ==
  Integrator : Integrator  ContinuousStateAttributes='Phase'
  Integrator1 : Integrator  ContinuousStateAttributes='Amplitude'
  Mux : Mux  Inputs=2
  Mux1 : Mux  Inputs=2
  Φ1_dot(t) : Subsystem
  α_dot(t) : Subsystem
  θ_estimated : Fcn  Expr=u(1)*sin(u(2))
  θ_est1 : Outport
  Phi_1 : Outport  Port=2
  tag scope: Alpha1_hip=global, Phi1_hip=global
  wires:
  Integrator/1 -> Mux/2, Phi_1/1, [Phi1_hip], Mux1/2  "Φ1(t)"
  Mux/1 -> Φ1_dot(t)/1(In1), α_dot(t)/1(Input)
  Integrator1/1 -> Mux/1, [Alpha1_hip], Mux1/1  "α1(t)"
  Mux1/1 -> θ_estimated/1
  θ_estimated/1 -> θ_est1/1  "θ_estimated"
  α_dot(t)/1(α_dot(t)) -> Integrator1/1
  Φ1_dot(t)/1(Φ1_dot(t)) -> Integrator/1

== system AOs_sim/Hip joint/(2) AOs3/AO2 ==
  Integrator : Integrator  ContinuousStateAttributes='Phase'
  Integrator1 : Integrator  ContinuousStateAttributes='Amplitude'
  Mux : Mux  Inputs=2
  Mux1 : Mux  Inputs=2
  Φ2_dot(t) : Subsystem
  α_dot(t) : Subsystem
  θ_estimated : Fcn  Expr=u(1)*sin(u(2))
  θ_est2 : Outport
  tag scope: Alpha2_hip=global
  wires:
  Integrator/1 -> Mux/2, Mux1/2  "Φ2(t)"
  Mux/1 -> Φ2_dot(t)/1(In1), α_dot(t)/1(Input)
  Integrator1/1 -> Mux/1, [Alpha2_hip], Mux1/1  "α2(t)"
  Mux1/1 -> θ_estimated/1
  θ_estimated/1 -> θ_est2/1  "θ_estimated"
  α_dot(t)/1(α_dot(t)) -> Integrator1/1
  Φ2_dot(t)/1(Φ2_dot(t)) -> Integrator/1

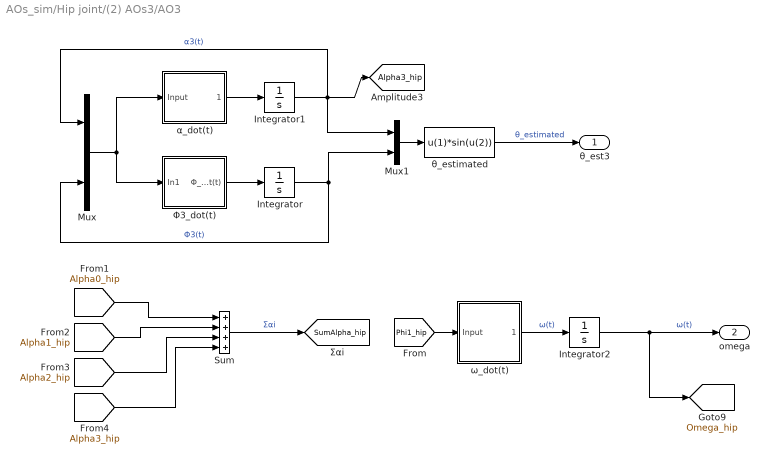
== system AOs_sim/Hip joint/(2) AOs3/AO3 ==
  Integrator : Integrator  ContinuousStateAttributes='Phase'
  Integrator1 : Integrator  ContinuousStateAttributes='Amplitude'
  Integrator2 : Integrator  UpperSaturationLimit=6*pi  LowerSaturationLimit=0  WrapState=on  WrappedStateUpperValue=10*pi  WrappedStateLowerValue=0  ContinuousStateAttributes='Omega'
  Mux : Mux  Inputs=2
  Mux1 : Mux  Inputs=2
  Sum : Sum  Inputs=++++
  Φ3_dot(t) : Subsystem
  α_dot(t) : Subsystem
  θ_estimated : Fcn  Expr=u(1)*sin(u(2))
  ω_dot(t) : Subsystem
  θ_est3 : Outport
  omega : Outport  Port=2
  tag scope: Alpha3_hip=global, Omega_hip=global, SumAlpha_hip=global
  wires:
  θ_estimated/1 -> θ_est3/1  "θ_estimated"
  α_dot(t)/1(α_dot(t)) -> Integrator1/1
  Integrator/1 -> Mux/2, Mux1/2  "Φ3(t)"
  Mux1/1 -> θ_estimated/1
  Φ3_dot(t)/1(Φ_dot(t)) -> Integrator/1
  Integrator1/1 -> Mux/1, [Alpha3_hip], Mux1/1  "α3(t)"
  Mux/1 -> Φ3_dot(t)/1(In1), α_dot(t)/1(Input)
  [Alpha1_hip] -> Sum/2
  [Alpha2_hip] -> Sum/3
  Sum/1 -> [SumAlpha_hip]  "Σαi"
  [Alpha3_hip] -> Sum/4
  [Alpha0_hip] -> Sum/1
  ω_dot(t)/1(ω_dot(t)) -> Integrator2/1  "ω(t)"
  [Phi1_hip] -> ω_dot(t)/1(Input)
  Integrator2/1 -> [Omega_hip], omega/1  "ω(t)"

== system AOs_sim/Hip joint/(3) Phase Error Compensation/Phase Error Calculator ==
  Φn : Inport
  tk : Inport  Port=2
  Constant : Constant
  Constant2 : Constant  Value=0
  Delay : Delay  DelayLength=1
  Memory : Memory
  Minus : Sum  Inputs=+-
  Subsystem : Subsystem
  Subsystem1 : Subsystem
  Switch : Switch  Criteria=u2 > Threshold  SaturateOnIntegerOverflow=off  InputSameDT=off
  Pe(tk) : Outport
  Pe_tilde(tk) : Outport  Port=2
  wires:
  Subsystem/1(Pe(tk)) -> Pe(tk)/1
  tk/1 -> Memory/1, Minus/1
  Memory/1 -> Minus/2
  Minus/1 -> Switch/2
  Constant2/1 -> Switch/3
  Constant/1 -> Switch/1
  Subsystem/2(Pe_tilde(tk)) -> Pe_tilde(tk)/1, Delay/1
  Φn/1 -> Subsystem/1(Φn)
  Subsystem1/1(Pe_tilde(tk-1)) -> Subsystem/2(Pe_tilde(tk-1))
  Switch/1 -> Subsystem1/Trigger, Subsystem/Trigger
  Delay/1 -> Subsystem1/1(Pe_tilde(tk))

== system AOs_sim/Hip joint/(3) Phase Error Compensation/Subsystem ==
  phi_e(t) : Inport
  Trigger : TriggerPort  VariantControl=Variant  PortDimensions=1
  phi_e(tk) : Outport
  wires:
  phi_e(t)/1 -> phi_e(tk)/1

== system AOs_sim/Knee joint/(1) Gait Event detector/Input derivative1 ==
  x : Inport
  Constant : Constant  Value=2
  Integrator1 : Integrator  InitialConditionSource=external
  Integrator2 : Integrator
  Product : Product  RndMeth=Zero
  Product1 : Product  RndMeth=Zero
  Product2 : Product  Inputs=3  RndMeth=Zero
  Sum : Sum  Inputs=|+-
  Sum1 : Sum  Inputs=|+-
  wn : Constant  Value=wn
  x0 : Constant  Value=x0
  zt : Constant  Value=zt
  y : Outport  VectorParamsAs1DForOutWhenUnconnected=off
  yd : Outport  Port=2  VectorParamsAs1DForOutWhenUnconnected=off
  wires:
  Sum/1 -> Product/2
  wn/1 -> Product/1, Product1/1
  Sum1/1 -> Sum/1
  x0/1 -> Integrator1/2
  Integrator2/1 -> Product1/2, Product2/1
  Product/1 -> Integrator2/1
  x/1 -> Sum1/1
  Product1/1 -> Integrator1/1, yd/1
  Integrator1/1 -> Sum1/2, y/1
  Product2/1 -> Sum/2
  zt/1 -> Product2/3
  Constant/1 -> Product2/2

== system AOs_sim/Knee joint/(1) Gait Event detector/t* detection ==
  clock : Inport
  Trigger : TriggerPort  VariantControl=Variant  PortDimensions=1
  t* : Outport
  wires:
  clock/1 -> t*/1

== system AOs_sim/Knee joint/(1) Gait Event detector/tk detection ==
  t* : Inport
  omega : Inport  Port=2
  tk-1 : Inport  Port=3
  Trigger : TriggerPort  VariantControl=Variant  PortDimensions=1
  Constant2 : Constant  Value=eps
  Constant3 : Constant  Value=2*pi
  Constant4 : Constant
  Constant5 : Constant  Value=0
  Divide : Product  Inputs=*/
  Minus : Sum  Inputs=+--
  Sum : Sum  Inputs=|++
  Switch1 : Switch  SaturateOnIntegerOverflow=off  InputSameDT=off
  ro : Gain  Gain=0.7
  tk+1 detection : Subsystem
  tk : Outport
  wires:
  Constant5/1 -> Switch1/3
  Sum/1 -> Divide/2
  Constant3/1 -> Divide/1
  Constant4/1 -> Switch1/1
  Constant2/1 -> Sum/2
  Divide/1 -> ro/1  "T(t)"
  t*/1 -> Minus/1, tk+1 detection/1(t*)
  tk-1/1 -> Minus/3
  ro/1 -> Minus/2
  tk+1 detection/1(tk) -> tk/1
  Switch1/1 -> tk+1 detection/Enable
  Minus/1 -> Switch1/2
  omega/1 -> Sum/1

== system AOs_sim/Knee joint/(2) AOs3/AO0 ==
  Integrator1 : Integrator  InitialCondition=0.01
  Product : Product
  α0 : Outport
  tag scope: Alpha0_knee=global
  wires:
  Product/1 -> Integrator1/1  "α0_dot(t)"
  [Eta_knee] -> Product/1
  [Ft_knee] -> Product/2
  Integrator1/1 -> [Alpha0_knee], α0/1  "α0(t)"

== system AOs_sim/Knee joint/(2) AOs3/AO1 ==
  Integrator : Integrator  ContinuousStateAttributes='Phase'
  Integrator1 : Integrator  ContinuousStateAttributes='Amplitude'
  Mux : Mux  Inputs=2
  Mux1 : Mux  Inputs=2
  Φ1_dot(t) : Subsystem
  α_dot(t) : Subsystem
  θ_estimated : Fcn  Expr=u(1)*sin(u(2))
  θ_est1 : Outport
  Phi_1 : Outport  Port=2
  tag scope: Alpha1_knee=global, Phi1_knee=global
  wires:
  Integrator/1 -> Mux/2, Phi_1/1, [Phi1_knee], Mux1/2  "Φ1(t)"
  Mux/1 -> Φ1_dot(t)/1(In1), α_dot(t)/1(Input)
  Integrator1/1 -> Mux/1, [Alpha1_knee], Mux1/1  "α1(t)"
  Mux1/1 -> θ_estimated/1
  θ_estimated/1 -> θ_est1/1  "θ_estimated"
  α_dot(t)/1(α_dot(t)) -> Integrator1/1
  Φ1_dot(t)/1(Φ1_dot(t)) -> Integrator/1

== system AOs_sim/Knee joint/(2) AOs3/AO2 ==
  Integrator : Integrator  ContinuousStateAttributes='Phase'
  Integrator1 : Integrator  ContinuousStateAttributes='Amplitude'
  Mux : Mux  Inputs=2
  Mux1 : Mux  Inputs=2
  Φ2_dot(t) : Subsystem
  α_dot(t) : Subsystem
  θ_estimated : Fcn  Expr=u(1)*sin(u(2))
  θ_est2 : Outport
  tag scope: Alpha2_knee=global
  wires:
  Integrator/1 -> Mux/2, Mux1/2  "Φ2(t)"
  Mux/1 -> Φ2_dot(t)/1(In1), α_dot(t)/1(Input)
  Integrator1/1 -> Mux/1, [Alpha2_knee], Mux1/1  "α2(t)"
  Mux1/1 -> θ_estimated/1
  θ_estimated/1 -> θ_est2/1  "θ_estimated"
  α_dot(t)/1(α_dot(t)) -> Integrator1/1
  Φ2_dot(t)/1(Φ2_dot(t)) -> Integrator/1

== system AOs_sim/Knee joint/(2) AOs3/AO3 ==
  Integrator : Integrator  ContinuousStateAttributes='Phase'
  Integrator1 : Integrator  ContinuousStateAttributes='Amplitude'
  Mux : Mux  Inputs=2
  Mux1 : Mux  Inputs=2
  Φ2_dot(t) : Subsystem
  α_dot(t) : Subsystem
  θ_estimated : Fcn  Expr=u(1)*sin(u(2))
  θ_est2 : Outport
  tag scope: Alpha3_knee=global
  wires:
  Integrator/1 -> Mux/2, Mux1/2  "Φ2(t)"
  Mux/1 -> Φ2_dot(t)/1(In1), α_dot(t)/1(Input)
  Integrator1/1 -> Mux/1, [Alpha3_knee], Mux1/1  "α2(t)"
  Mux1/1 -> θ_estimated/1
  θ_estimated/1 -> θ_est2/1  "θ_estimated"
  α_dot(t)/1(α_dot(t)) -> Integrator1/1
  Φ2_dot(t)/1(Φ2_dot(t)) -> Integrator/1

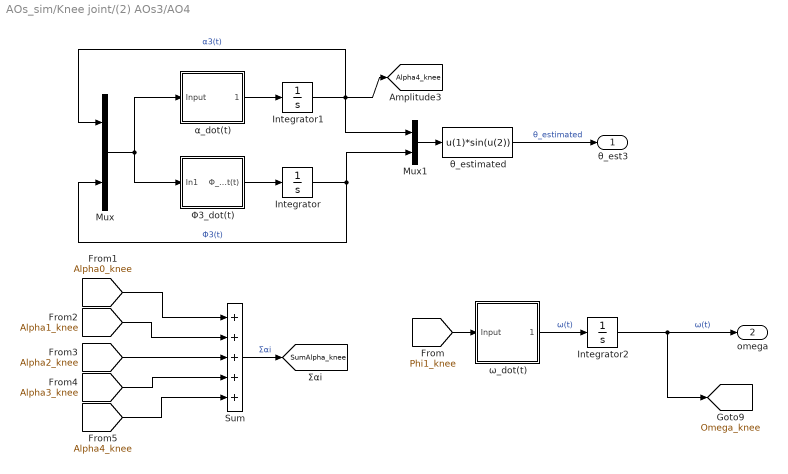
== system AOs_sim/Knee joint/(2) AOs3/AO4 ==
  Integrator : Integrator  ContinuousStateAttributes='Phase'
  Integrator1 : Integrator  ContinuousStateAttributes='Amplitude'
  Integrator2 : Integrator  WrapState=on  WrappedStateUpperValue=10*pi  WrappedStateLowerValue=0  ContinuousStateAttributes='Omega'
  Mux : Mux  Inputs=2
  Mux1 : Mux  Inputs=2
  Sum : Sum  Inputs=+++++
  Φ3_dot(t) : Subsystem
  α_dot(t) : Subsystem
  θ_estimated : Fcn  Expr=u(1)*sin(u(2))
  ω_dot(t) : Subsystem
  θ_est3 : Outport
  omega : Outport  Port=2
  tag scope: Alpha4_knee=global, Omega_knee=global, SumAlpha_knee=global
  wires:
  θ_estimated/1 -> θ_est3/1  "θ_estimated"
  α_dot(t)/1(α_dot(t)) -> Integrator1/1
  Integrator/1 -> Mux/2, Mux1/2  "Φ3(t)"
  Mux1/1 -> θ_estimated/1
  Φ3_dot(t)/1(Φ_dot(t)) -> Integrator/1
  Integrator1/1 -> Mux/1, [Alpha4_knee], Mux1/1  "α3(t)"
  Mux/1 -> Φ3_dot(t)/1(In1), α_dot(t)/1(Input)
  [Alpha1_knee] -> Sum/2
  [Alpha2_knee] -> Sum/3
  Sum/1 -> [SumAlpha_knee]  "Σαi"
  [Alpha3_knee] -> Sum/4
  [Alpha0_knee] -> Sum/1
  ω_dot(t)/1(ω_dot(t)) -> Integrator2/1  "ω(t)"
  [Phi1_knee] -> ω_dot(t)/1(Input)
  Integrator2/1 -> [Omega_knee], omega/1  "ω(t)"
  [Alpha4_knee] -> Sum/5

== system AOs_sim/Knee joint/(3) Phase Error Compensation/Phase Error Calculator ==
  Φn : Inport
  tk : Inport  Port=2
  Constant : Constant
  Constant2 : Constant  Value=0
  Delay : Delay  DelayLength=1
  Memory : Memory
  Minus : Sum  Inputs=+-
  Subsystem : Subsystem
  Subsystem1 : Subsystem
  Switch : Switch  Criteria=u2 > Threshold  SaturateOnIntegerOverflow=off  InputSameDT=off
  Pe(tk) : Outport
  Pe_tilde(tk) : Outport  Port=2
  wires:
  Subsystem/1(Pe(tk)) -> Pe(tk)/1
  tk/1 -> Memory/1, Minus/1
  Memory/1 -> Minus/2
  Minus/1 -> Switch/2
  Constant2/1 -> Switch/3
  Constant/1 -> Switch/1
  Subsystem/2(Pe_tilde(tk)) -> Pe_tilde(tk)/1, Delay/1
  Φn/1 -> Subsystem/1(Φn)
  Subsystem1/1(Pe_tilde(tk-1)) -> Subsystem/2(Pe_tilde(tk-1))
  Switch/1 -> Subsystem1/Trigger, Subsystem/Trigger
  Delay/1 -> Subsystem1/1(Pe_tilde(tk))

== system AOs_sim/Knee joint/(3) Phase Error Compensation/Subsystem ==
  phi_e(t) : Inport
  Trigger : TriggerPort  VariantControl=Variant  PortDimensions=1
  phi_e(tk) : Outport
  wires:
  phi_e(t)/1 -> phi_e(tk)/1

== system AOs_sim/Ankle joint/(1) Gait Event detector/tk detection/tk+1 detection ==
  t* : Inport
  Enable : EnablePort
  tk : Outport
  wires:
  t*/1 -> tk/1

== system AOs_sim/Ankle joint/(2) AOs4/AO1/Φ1_dot(t) ==
  In1 : Inport
  Constant : Constant
  Divide : Product  Inputs=*/
  Product : Product  Inputs=3
  Product1 : Product
  Sum : Sum
  Sum1 : Sum
  cos(Φ1(t)) : Fcn  Expr=cos(u(2))
  Φ1_dot(t) : Outport
  wires:
  Sum/1 -> Φ1_dot(t)/1
  In1/1 -> cos(Φ1(t))/1
  [vphi_ankle] -> Product/1
  cos(Φ1(t))/1 -> Product/3
  Product/1 -> Sum/2
  Constant/1 -> Product1/1
  [Omega_ankle] -> Product1/2
  Product1/1 -> Sum/1
  [Ft_ankle] -> Divide/1
  Sum1/1 -> Divide/2
  Divide/1 -> Product/2
  [Alpha1_ankle] -> Sum1/2
  [Alpha0_ankle] -> Sum1/1

== system AOs_sim/Ankle joint/(2) AOs4/AO1/α_dot(t) ==
  Input : Inport
  Product : Product  Inputs=3
  α_dot : Fcn  Expr=sin(u(2))
  α_dot(t) : Outport
  wires:
  Product/1 -> α_dot(t)/1
  [Eta_ankle] -> Product/1
  α_dot/1 -> Product/3
  [Ft_ankle] -> Product/2
  Input/1 -> α_dot/1

== system AOs_sim/Ankle joint/(2) AOs4/AO2/Φ2_dot(t) ==
  In1 : Inport
  Constant : Constant  Value=2
  Divide : Product  Inputs=*/
  Product : Product  Inputs=3
  Product1 : Product
  Sum : Sum
  Sum1 : Sum  Inputs=+++
  cos(Φ2(t)) : Fcn  Expr=cos(u(2))
  Φ2_dot(t) : Outport
  wires:
  Sum/1 -> Φ2_dot(t)/1
  In1/1 -> cos(Φ2(t))/1
  [vphi_ankle] -> Product/1
  cos(Φ2(t))/1 -> Product/3
  Product/1 -> Sum/2
  Constant/1 -> Product1/1
  [Omega_ankle] -> Product1/2
  Product1/1 -> Sum/1
  [Ft_ankle] -> Divide/1
  Sum1/1 -> Divide/2
  Divide/1 -> Product/2
  [Alpha0_ankle] -> Sum1/1
  [Alpha2_ankle] -> Sum1/3
  [Alpha1_ankle] -> Sum1/2

== system AOs_sim/Ankle joint/(2) AOs4/AO2/α_dot(t) ==
  Input : Inport
  Product : Product  Inputs=3
  sin(Φ2(t)) : Fcn  Expr=sin(u(2))
  α_dot(t) : Outport
  wires:
  Product/1 -> α_dot(t)/1
  [Eta_ankle] -> Product/1
  sin(Φ2(t))/1 -> Product/3
  [Ft_ankle] -> Product/2
  Input/1 -> sin(Φ2(t))/1

== system AOs_sim/Ankle joint/(2) AOs4/AO3/Φ2_dot(t) ==
  In1 : Inport
  Constant : Constant  Value=2
  Divide : Product  Inputs=*/
  Product : Product  Inputs=3
  Product1 : Product
  Sum : Sum
  Sum1 : Sum  Inputs=++++
  cos(Φ2(t)) : Fcn  Expr=cos(u(2))
  Φ2_dot(t) : Outport
  wires:
  Sum/1 -> Φ2_dot(t)/1
  In1/1 -> cos(Φ2(t))/1
  [vphi_ankle] -> Product/1
  cos(Φ2(t))/1 -> Product/3
  Product/1 -> Sum/2
  Constant/1 -> Product1/1
  [Omega_ankle] -> Product1/2
  Product1/1 -> Sum/1
  [Ft_ankle] -> Divide/1
  Sum1/1 -> Divide/2
  Divide/1 -> Product/2
  [Alpha0_ankle] -> Sum1/1
  [Alpha2_ankle] -> Sum1/3
  [Alpha1_ankle] -> Sum1/2
  [Alpha3_ankle] -> Sum1/4

== system AOs_sim/Ankle joint/(2) AOs4/AO3/α_dot(t) ==
  Input : Inport
  Product : Product  Inputs=3
  sin(Φ2(t)) : Fcn  Expr=sin(u(2))
  α_dot(t) : Outport
  wires:
  Product/1 -> α_dot(t)/1
  [Eta_ankle] -> Product/1
  sin(Φ2(t))/1 -> Product/3
  [Ft_ankle] -> Product/2
  Input/1 -> sin(Φ2(t))/1

== system AOs_sim/Ankle joint/(2) AOs4/AO4/Φ3_dot(t) ==
  In1 : Inport
  Constant : Constant  Value=3
  Divide : Product  Inputs=*/
  Product : Product  Inputs=3
  Product1 : Product
  Sum : Sum
  cos(Φ(t)) : Fcn  Expr=cos(u(2))
  Φ_dot(t) : Outport
  wires:
  Divide/1 -> Product/2
  Sum/1 -> Φ_dot(t)/1
  In1/1 -> cos(Φ(t))/1
  [vphi_ankle] -> Product/1
  cos(Φ(t))/1 -> Product/3
  Product/1 -> Sum/2
  Constant/1 -> Product1/1
  [Omega_ankle] -> Product1/2
  Product1/1 -> Sum/1
  [Ft_ankle] -> Divide/1
  [SumAlpha_ankle] -> Divide/2

== system AOs_sim/Ankle joint/(2) AOs4/AO4/α_dot(t) ==
  Input : Inport
  Product : Product  Inputs=3
  sin(Φ3(t)) : Fcn  Expr=sin(u(2))
  α_dot(t) : Outport
  wires:
  Product/1 -> α_dot(t)/1
  [Eta_ankle] -> Product/1
  sin(Φ3(t))/1 -> Product/3
  [Ft_ankle] -> Product/2
  Input/1 -> sin(Φ3(t))/1

== system AOs_sim/Ankle joint/(2) AOs4/AO4/ω_dot(t) ==
  Input : Inport
  Divide : Product  Inputs=*/
  Product : Product  Inputs=3
  cos(Φ1(t)) : Fcn  Expr=cos(u(1))
  ω_dot(t) : Outport
  wires:
  Product/1 -> ω_dot(t)/1
  [vomega_ankle] -> Product/1
  Input/1 -> cos(Φ1(t))/1
  cos(Φ1(t))/1 -> Product/3
  [Ft_ankle] -> Divide/1
  Divide/1 -> Product/2
  [SumAlpha_ankle] -> Divide/2

== system AOs_sim/Ankle joint/(2) AOs4/AO5/Φ2_dot(t) ==
  In1 : Inport
  Constant : Constant  Value=2
  Divide : Product  Inputs=*/
  Product : Product  Inputs=3
  Product1 : Product
  Sum : Sum
  Sum1 : Sum  Inputs=+++++
  cos(Φ2(t)) : Fcn  Expr=cos(u(2))
  Φ2_dot(t) : Outport
  wires:
  Sum/1 -> Φ2_dot(t)/1
  In1/1 -> cos(Φ2(t))/1
  [vphi_ankle] -> Product/1
  cos(Φ2(t))/1 -> Product/3
  Product/1 -> Sum/2
  Constant/1 -> Product1/1
  [Omega_ankle] -> Product1/2
  Product1/1 -> Sum/1
  [Ft_ankle] -> Divide/1
  Sum1/1 -> Divide/2
  Divide/1 -> Product/2
  [Alpha0_ankle] -> Sum1/1
  [Alpha2_ankle] -> Sum1/3
  [Alpha1_ankle] -> Sum1/2
  [Alpha3_ankle] -> Sum1/4
  [Alpha4_ankle] -> Sum1/5

== system AOs_sim/Ankle joint/(2) AOs4/AO5/α_dot(t) ==
  Input : Inport
  Product : Product  Inputs=3
  sin(Φ2(t)) : Fcn  Expr=sin(u(2))
  α_dot(t) : Outport
  wires:
  Product/1 -> α_dot(t)/1
  [Eta_ankle] -> Product/1
  sin(Φ2(t))/1 -> Product/3
  [Ft_ankle] -> Product/2
  Input/1 -> sin(Φ2(t))/1

== system AOs_sim/Ankle joint/(3) Phase Error Compensation/Phase Error Calculator/Subsystem ==
  Φn : Inport
  Pe_tilde(tk-1) : Inport  Port=2
  Trigger : TriggerPort  VariantControl=Variant  PortDimensions=1
  PE : Subsystem
  PE Further Updated : Subsystem
  Pe(tk) : Outport
  Pe_tilde(tk) : Outport  Port=2
  wires:
  PE/1(Pe(tk)) -> PE Further Updated/1(Pe(tk)), Pe(tk)/1
  PE Further Updated/1(Pe_tilde(tk)) -> Pe_tilde(tk)/1
  Pe_tilde(tk-1)/1 -> PE Further Updated/2(Pe_tilde(tk-1))
  Φn/1 -> PE/1(Φn(tk))

== system AOs_sim/Ankle joint/(3) Phase Error Compensation/Phase Error Calculator/Subsystem1 ==
  Pe_tilde(tk) : Inport
  Trigger : TriggerPort  VariantControl=Variant  PortDimensions=1
  Pe_tilde(tk-1) : Outport
  wires:
  Pe_tilde(tk)/1 -> Pe_tilde(tk-1)/1

== system AOs_sim/Hip joint/(1) Gait Event detector/tk detection/tk+1 detection ==
  t* : Inport
  Enable : EnablePort
  tk : Outport
  wires:
  t*/1 -> tk/1

== system AOs_sim/Hip joint/(2) AOs3/AO1/Φ1_dot(t) ==
  In1 : Inport
  Constant : Constant
  Divide : Product  Inputs=*/
  Product : Product  Inputs=3
  Product1 : Product
  Sum : Sum
  Sum1 : Sum
  cos(Φ1(t)) : Fcn  Expr=cos(u(2))
  Φ1_dot(t) : Outport
  wires:
  Sum/1 -> Φ1_dot(t)/1
  In1/1 -> cos(Φ1(t))/1
  [vphi_hip] -> Product/1
  cos(Φ1(t))/1 -> Product/3
  Product/1 -> Sum/2
  Constant/1 -> Product1/1
  [Omega_hip] -> Product1/2
  Product1/1 -> Sum/1
  [Ft_hip] -> Divide/1
  Sum1/1 -> Divide/2
  Divide/1 -> Product/2
  [Alpha1_hip] -> Sum1/2
  [Alpha0_hip] -> Sum1/1

== system AOs_sim/Hip joint/(2) AOs3/AO1/α_dot(t) ==
  Input : Inport
  Product : Product  Inputs=3
  α_dot : Fcn  Expr=sin(u(2))
  α_dot(t) : Outport
  wires:
  Product/1 -> α_dot(t)/1
  [Eta_hip] -> Product/1
  α_dot/1 -> Product/3
  [Ft_hip] -> Product/2
  Input/1 -> α_dot/1

== system AOs_sim/Hip joint/(2) AOs3/AO2/Φ2_dot(t) ==
  In1 : Inport
  Constant : Constant  Value=2
  Divide : Product  Inputs=*/
  Product : Product  Inputs=3
  Product1 : Product
  Sum : Sum
  Sum1 : Sum  Inputs=+++
  cos(Φ2(t)) : Fcn  Expr=cos(u(2))
  Φ2_dot(t) : Outport
  wires:
  Sum/1 -> Φ2_dot(t)/1
  In1/1 -> cos(Φ2(t))/1
  [vphi_hip] -> Product/1
  cos(Φ2(t))/1 -> Product/3
  Product/1 -> Sum/2
  Constant/1 -> Product1/1
  [Omega_hip] -> Product1/2
  Product1/1 -> Sum/1
  [Ft_hip] -> Divide/1
  Sum1/1 -> Divide/2
  Divide/1 -> Product/2
  [Alpha0_hip] -> Sum1/1
  [Alpha2_hip] -> Sum1/3
  [Alpha1_hip] -> Sum1/2

== system AOs_sim/Hip joint/(2) AOs3/AO2/α_dot(t) ==
  Input : Inport
  Product : Product  Inputs=3
  sin(Φ2(t)) : Fcn  Expr=sin(u(2))
  α_dot(t) : Outport
  wires:
  Product/1 -> α_dot(t)/1
  [Eta_hip] -> Product/1
  sin(Φ2(t))/1 -> Product/3
  [Ft_hip] -> Product/2
  Input/1 -> sin(Φ2(t))/1

== system AOs_sim/Hip joint/(2) AOs3/AO3/Φ3_dot(t) ==
  In1 : Inport
  Constant : Constant  Value=3
  Divide : Product  Inputs=*/
  Product : Product  Inputs=3
  Product1 : Product
  Sum : Sum
  cos(Φ(t)) : Fcn  Expr=cos(u(2))
  Φ_dot(t) : Outport
  wires:
  Divide/1 -> Product/2
  Sum/1 -> Φ_dot(t)/1
  In1/1 -> cos(Φ(t))/1
  [vphi_hip] -> Product/1
  cos(Φ(t))/1 -> Product/3
  Product/1 -> Sum/2
  Constant/1 -> Product1/1
  [Omega_hip] -> Product1/2
  Product1/1 -> Sum/1
  [Ft_hip] -> Divide/1
  [SumAlpha_hip] -> Divide/2

== system AOs_sim/Hip joint/(2) AOs3/AO3/α_dot(t) ==
  Input : Inport
  Product : Product  Inputs=3
  sin(Φ3(t)) : Fcn  Expr=sin(u(2))
  α_dot(t) : Outport
  wires:
  Product/1 -> α_dot(t)/1
  [Eta_hip] -> Product/1
  sin(Φ3(t))/1 -> Product/3
  [Ft_hip] -> Product/2
  Input/1 -> sin(Φ3(t))/1

== system AOs_sim/Hip joint/(2) AOs3/AO3/ω_dot(t) ==
  Input : Inport
  Divide : Product  Inputs=*/
  Product : Product  Inputs=3
  cos(Φ1(t)) : Fcn  Expr=cos(u(1))
  ω_dot(t) : Outport
  wires:
  Product/1 -> ω_dot(t)/1
  [vomega_hip] -> Product/1
  Input/1 -> cos(Φ1(t))/1
  cos(Φ1(t))/1 -> Product/3
  [Ft_hip] -> Divide/1
  Divide/1 -> Product/2
  [SumAlpha_hip] -> Divide/2

== system AOs_sim/Hip joint/(3) Phase Error Compensation/Phase Error Calculator/Subsystem ==
  Φn : Inport
  Pe_tilde(tk-1) : Inport  Port=2
  Trigger : TriggerPort  VariantControl=Variant  PortDimensions=1
  PE : Subsystem
  PE Further Updated : Subsystem
  Pe(tk) : Outport
  Pe_tilde(tk) : Outport  Port=2
  wires:
  PE/1(Pe(tk)) -> PE Further Updated/1(Pe(tk)), Pe(tk)/1
  PE Further Updated/1(Pe_tilde(tk)) -> Pe_tilde(tk)/1
  Pe_tilde(tk-1)/1 -> PE Further Updated/2(Pe_tilde(tk-1))
  Φn/1 -> PE/1(Φn(tk))

== system AOs_sim/Hip joint/(3) Phase Error Compensation/Phase Error Calculator/Subsystem1 ==
  Pe_tilde(tk) : Inport
  Trigger : TriggerPort  VariantControl=Variant  PortDimensions=1
  Pe_tilde(tk-1) : Outport
  wires:
  Pe_tilde(tk)/1 -> Pe_tilde(tk-1)/1

== system AOs_sim/Knee joint/(1) Gait Event detector/tk detection/tk+1 detection ==
  t* : Inport
  Enable : EnablePort
  tk : Outport
  wires:
  t*/1 -> tk/1

== system AOs_sim/Knee joint/(2) AOs3/AO1/Φ1_dot(t) ==
  In1 : Inport
  Constant : Constant
  Divide : Product  Inputs=*/
  Product : Product  Inputs=3
  Product1 : Product
  Sum : Sum
  Sum1 : Sum
  cos(Φ1(t)) : Fcn  Expr=cos(u(2))
  Φ1_dot(t) : Outport
  wires:
  Sum/1 -> Φ1_dot(t)/1
  In1/1 -> cos(Φ1(t))/1
  [vphi_knee] -> Product/1
  cos(Φ1(t))/1 -> Product/3
  Product/1 -> Sum/2
  Constant/1 -> Product1/1
  [Omega_knee] -> Product1/2
  Product1/1 -> Sum/1
  [Ft_knee] -> Divide/1
  Sum1/1 -> Divide/2
  Divide/1 -> Product/2
  [Alpha1_knee] -> Sum1/2
  [Alpha0_knee] -> Sum1/1

== system AOs_sim/Knee joint/(2) AOs3/AO1/α_dot(t) ==
  Input : Inport
  Product : Product  Inputs=3
  α_dot : Fcn  Expr=sin(u(2))
  α_dot(t) : Outport
  wires:
  Product/1 -> α_dot(t)/1
  [Eta_knee] -> Product/1
  α_dot/1 -> Product/3
  [Ft_knee] -> Product/2
  Input/1 -> α_dot/1

== system AOs_sim/Knee joint/(2) AOs3/AO2/Φ2_dot(t) ==
  In1 : Inport
  Constant : Constant  Value=2
  Divide : Product  Inputs=*/
  Product : Product  Inputs=3
  Product1 : Product
  Sum : Sum
  Sum1 : Sum  Inputs=+++
  cos(Φ2(t)) : Fcn  Expr=cos(u(2))
  Φ2_dot(t) : Outport
  wires:
  Sum/1 -> Φ2_dot(t)/1
  In1/1 -> cos(Φ2(t))/1
  [vphi_knee] -> Product/1
  cos(Φ2(t))/1 -> Product/3
  Product/1 -> Sum/2
  Constant/1 -> Product1/1
  [Omega_knee] -> Product1/2
  Product1/1 -> Sum/1
  [Ft_knee] -> Divide/1
  Sum1/1 -> Divide/2
  Divide/1 -> Product/2
  [Alpha0_knee] -> Sum1/1
  [Alpha2_knee] -> Sum1/3
  [Alpha1_knee] -> Sum1/2

== system AOs_sim/Knee joint/(2) AOs3/AO2/α_dot(t) ==
  Input : Inport
  Product : Product  Inputs=3
  sin(Φ2(t)) : Fcn  Expr=sin(u(2))
  α_dot(t) : Outport
  wires:
  Product/1 -> α_dot(t)/1
  [Eta_knee] -> Product/1
  sin(Φ2(t))/1 -> Product/3
  [Ft_knee] -> Product/2
  Input/1 -> sin(Φ2(t))/1

== system AOs_sim/Knee joint/(2) AOs3/AO3/Φ2_dot(t) ==
  In1 : Inport
  Constant : Constant  Value=2
  Divide : Product  Inputs=*/
  Product : Product  Inputs=3
  Product1 : Product
  Sum : Sum
  Sum1 : Sum  Inputs=++++
  cos(Φ2(t)) : Fcn  Expr=cos(u(2))
  Φ2_dot(t) : Outport
  wires:
  Sum/1 -> Φ2_dot(t)/1
  In1/1 -> cos(Φ2(t))/1
  [vphi_knee] -> Product/1
  cos(Φ2(t))/1 -> Product/3
  Product/1 -> Sum/2
  Constant/1 -> Product1/1
  [Omega_knee] -> Product1/2
  Product1/1 -> Sum/1
  [Ft_knee] -> Divide/1
  Sum1/1 -> Divide/2
  Divide/1 -> Product/2
  [Alpha0_knee] -> Sum1/1
  [Alpha2_knee] -> Sum1/3
  [Alpha1_knee] -> Sum1/2
  [Alpha3_knee] -> Sum1/4

== system AOs_sim/Knee joint/(2) AOs3/AO3/α_dot(t) ==
  Input : Inport
  Product : Product  Inputs=3
  sin(Φ2(t)) : Fcn  Expr=sin(u(2))
  α_dot(t) : Outport
  wires:
  Product/1 -> α_dot(t)/1
  [Eta_knee] -> Product/1
  sin(Φ2(t))/1 -> Product/3
  [Ft_knee] -> Product/2
  Input/1 -> sin(Φ2(t))/1
